simulink model "x35BusNetworkElectricityTransmissionModel"  (R2023b)
settings: Solver=VariableStepAuto  StartTime=0.0  StopTime=0.8  RelTol=1e-3
model workspace (MAT data in the model file):
  Compensation_Ki = 30
  Compensation_Kp = 3
  DC_Ki = 400
  DC_Kp = 8
  F = 0.01
  Flux_min = 0.5
  Grid_Freq_PWM = 2700
  Grid_Ireg_Ki = 5
  Grid_Ireg_Kp = 0.83
  Grid_Ireg_lim = 1.1
  Grid_Modindex_Upper = 1.1
  Grid_conv_Imax = 0.8
  H = 0.685
  Idref_max = 0.9
  Iqref_Tc = 0.3
  Ki_Var = 0.05
  Ki_Vreg = 20
  Ksh = 1.1
  L_pu = 0.3
  Llr = 0.16
  Lls = 0.18
  Lm = 2.9
  Nb_wt = 6
  P_mech = 1080000
  Pitch_Ki = 0
  Pitch_Kp = 150
  Pitch_Max = 27
  Pitch_Tc = 0.01
  Pitch_rate = 10
  Q_Filt = 50
  R_pu = 0.003
  Rotor_Freq_PWM = 1620
  Rotor_Ireg_Ki = 8
  Rotor_Ireg_Kp = 0.6
  Rotor_Ireg_lim = 0.1
  Rotor_Modindex_Upper = 2
  Rr = 0.016
  Rs = 0.023
  T_set = 0.0001
  Tp = 5e-05
  Ts = 5e-06
  Var_C_Filt = 720000
  Var_reg_max = 1.1
  Var_reg_min = 0.9
  WT_Coeff = [0.645 116 0.4 5 21 0.00912 0.08 0.035]
  WT_H = 4.32
  WT_IGBTRon = 5.931
  WT_Param = [91.204 10143]
  Wind_Freq_Filt = 10000
  Wind_Freq_nom = 60
  Wind_P_nom = 1200000
  Wind_Rotor_V_nom = 1950
  Wind_V_nom = 500
  Zeta_Filt = 0.707106781187
  init = [-0.2 0 0 0 0 0 0 0]
  p = 3
  torque0 = 0.83
  v_Ki = 0.1
  v_Kp = 3.6
  v_Max = 1.2
  v_Min = 0.7
  v_T = 5
  vreg_max = 1
  wind_VDC_nom = 1150
  wt0 = 1.2
undefined symbols (not defined in the file): D1, D11, Delta, DiscIntNeverNeededParam, Ion, Lithium, P, Q
libraries: powerlib_extras x144, spsSeriesRLCBranchLib x67, spsLoadFlowBusLib x43, spsThreePhaseTransformerTwoWindingsLib x32, spsThreePhaseSeriesRLCLoadLib x31, spsThreePhaseVIMeasurementLib x26, simulink_extras x26, spsDistributedParametersLineLib x22, spsGenericPowerSystemStabilizerLib x20, spsSynchronousMachinepuStandardLib x10, spsExcitationSystemLib x10, spsHydraulicTurbineandGovernorLib x10
(part 8 of 16)

== system x35BusNetworkElectricityTransmissionModel/400 kV Solar Farm/VSC Control/Current Regulator ==
  VdVq_mes : Inport  PortDimensions=2
  IdIq_mes : Inport  Port=2  PortDimensions=2
  IdIq_ref : Inport  Port=3  PortDimensions=2
  Add1 : Sum  Inputs=++-
  Add2 : Sum
  Add3 : Sum  Inputs=+++
  Demux : Demux  Outputs=2
  Demux1 : Demux  Outputs=2
  Ltot_pu1 : Gain  Gain=Ltot_pu  SaturateOnIntegerOverflow=on  OutDataTypeStr=Inherit: Same as input  ParamDataTypeStr=Inherit: Same as input
  Ltot_pu2 : Gain  Gain=Ltot_pu  SaturateOnIntegerOverflow=on  OutDataTypeStr=Inherit: Same as input  ParamDataTypeStr=Inherit: Same as input
  Mux : Mux  Inputs=2
  PI : slpidlib/PID Controller  Controller=PI  Form=Parallel  TimeDomain=Discrete-time  UseExternalTs=off  SampleTime=Ts  IntegratorMethod=Forward Euler  FilterMethod=Forward Euler  ControllerParametersSource=internal  P=Kp_Ireg  I=Ki_Ireg  UseKiTs=off  D=0  N=100  UseFilter=on  TunerSelectOption=Transfer Function Based (PID Tuner App)  InitialConditionSource=internal  InitialConditionForIntegrator=0  InitialConditionForFilter=0  DifferentiatorICPrevScaledInput=0  ExternalReset=none  TrackingMode=off  Kt=1  LimitOutput=on  SatLimitsSource=internal  UpperSaturationLimit=2  LowerSaturationLimit=-2  LinearizeAsGain=off  AntiWindupMode=none  Kb=1  LimitIntegrator=off  UpperIntegratorSaturationLimit=inf  LowerIntegratorSaturationLimit=-inf  POutMin=[]  POutMax=[]  IOutMin=[]  IOutMax=[]  DOutMin=[]  DOutMax=[]  NOutMin=[]  NOutMax=[]  SumOutMin=[]  SumOutMax=[]  SaturationOutMin=[]  SaturationOutMax=[]  PParamMin=[]  PParamMax=[]  IParamMin=[]  IParamMax=[]  DParamMin=[]  DParamMax=[]  NParamMin=[]  NParamMax=[]  KbParamMin=[]  KbParamMax=[]  KtParamMin=[]  KtParamMax=[]  KbOutMin=[]  KbOutMax=[]  KtOutMin=[]  KtOutMax=[]  IntegratorOutMin=[]  IntegratorOutMax=[]  FilterOutMin=[]  FilterOutMax=[]  SumI1OutMin=[]  SumI1OutMax=[]  SumI2OutMin=[]  SumI2OutMax=[]  SumI3OutMin=[]  SumI3OutMax=[]  SumI4OutMin=[]  SumI4OutMax=[]  SumDOutMin=[]  SumDOutMax=[]  DifferentiatorOutMin=[]  DifferentiatorOutMax=[]  FilterDiffOutCoefMin=[]  FilterDiffOutCoefMax=[]  ReciprocalOutMin=[]  ReciprocalOutMax=[]  SumDenOutMin=[]  SumDenOutMax=[]  SumNumOutMin=[]  SumNumOutMax=[]  DivideOutMin=[]  DivideOutMax=[]  UdiffTsProdOutMin=[]  UdiffTsProdOutMax=[]  NTsProdOutMin=[]  NTsProdOutMax=[]  UintegralTsProdOutMin=[]  UintegralTsProdOutMax=[]  UngainTsProdOutMin=[]  UngainTsProdOutMax=[]  ClampingZeroOutDataTypeStr=Inherit: Inherit via back propagation  ClampingZeroOutMin=[]  ClampingZeroOutMax=[]  FilterDenConstantOutDataTypeStr=Inherit: Inherit via back propagation  FilterDenConstantOutMin=[]  FilterDenConstantOutMax=[]  PCopyOutDataTypeStr=Inherit: Inherit via back propagation  PCopyOutMin=[]  PCopyOutMax=[]  NCopyOutDataTypeStr=Inherit: Inherit via back propagation  NCopyOutMin=[]  NCopyOutMax=[]  IntegratorContinuousStateAttributes=''  IntegratorStateMustResolveToSignalObject=off  IntegratorRTWStateStorageClass=Auto  FilterContinuousStateAttributes=''  FilterStateMustResolveToSignalObject=off  FilterRTWStateStorageClass=Auto  ParallelPVariant=InternalParameters  IdealPVariant=Disabled  IVariant=InternalParameters  DVariant=Disabled  IntegratorVariant=Discrete  SatVariant=Enabled  AWVariant=Passthrough  PCopyVariant=Disabled  TRVariant=Disabled  FdbkBlocksVariant=Forward  IdealPFdbkVariant=Disabled  SatFdbkVariant=Disabled  DerivativeFilterVariant=Disabled  NVariant=Disabled  NCopyVariant=Disabled_SignalSpec  FilterICVariant=Disabled  IntegratorICVariant=InternalICs  ExternalResetVariant=Disabled  TRSumVariant=Passthrough  SumFdbkVariant=Disabled  SumVariant=Sum_PI  TsampFilterVariant=InternalTs  TsampNgainVariant=Passthrough  TsampIntegralVariant=Disabled_SignalSpec  ExternalSaturationOutDataTypeStr=Inherit: Same as second input
  PI_Ireg1 : Scope
  Rtot_pu1 : Gain  Gain=Rtot_pu  SaturateOnIntegerOverflow=on  OutDataTypeStr=Inherit: Same as input  ParamDataTypeStr=Inherit: Same as input
  Rtot_pu5 : Gain  Gain=Rtot_pu  SaturateOnIntegerOverflow=on  OutDataTypeStr=Inherit: Same as input  ParamDataTypeStr=Inherit: Same as input
  Saturation : Saturate  UpperLimit=2  LowerLimit=-2
  Sum : Sum  Inputs=|-+
  VdVq_conv : Outport  VectorParamsAs1DForOutWhenUnconnected=off
  wires:
  Mux/1 -> PI_Ireg1/1, Add2/2
  PI/1 -> Add2/1  "PI"
  Sum/1 -> PI/1
  IdIq_ref/1 -> Sum/2, Demux1/1
  IdIq_mes/1 -> Sum/1
  Add2/1 -> Saturation/1
  Saturation/1 -> VdVq_conv/1
  VdVq_mes/1 -> Demux/1
  Demux/1 -> Add1/1
  Rtot_pu1/1 -> Add1/2
  Demux1/1 -> Rtot_pu1/1, Ltot_pu2/1
  Ltot_pu1/1 -> Add1/3
  Demux1/2 -> Ltot_pu1/1, Rtot_pu5/1
  Rtot_pu5/1 -> Add3/2
  Ltot_pu2/1 -> Add3/3
  Add1/1 -> Mux/1  "Feedforward"
  Demux/2 -> Add3/1
  Add3/1 -> Mux/2

== system x35BusNetworkElectricityTransmissionModel/400 kV Solar Farm/VSC Control/PLL & Measurements ==
  Vabc_prim : Inport
  Iabc_prim : Inport  Port=2
  PLL (3ph) : spsPLL3phLib/PLL (3ph)  Fmin=45  Par_Init="[-0.57  Fnom]"  ParK=[180, 3200, 1]  TcD=Ts  MaxRateChangeFreq=12  FilterCutOffFreq=25  Ts=Ts  AGC=on
  Selector1 : Selector  InputPortWidth=3  IndexOptions=Index vector (dialog)  Indices=[1 2]  OutputSizes=1
  Selector2 : Selector  InputPortWidth=3  IndexOptions=Index vector (dialog)  Indices=[1 2]  OutputSizes=1
  Terminator : Terminator
  V->pu : Gain  Gain=1/(Vnom_prim*sqrt(2)/sqrt(3))  SaturateOnIntegerOverflow=on  OutDataTypeStr=Inherit: Same as input  ParamDataTypeStr=Inherit: Same as input
  V->pu1 : Gain  Gain=Vnom_prim*sqrt(3)/Pnom/sqrt(2)  SaturateOnIntegerOverflow=on  OutDataTypeStr=Inherit: Same as input  ParamDataTypeStr=Inherit: Same as input
  abc to dq0 : spsabctodq0Lib/abc to dq0  Alignment=90 degrees behind phase A axis
  abc to dq1 : spsabctodq0Lib/abc to dq0  Alignment=90 degrees behind phase A axis
  wt : Outport  VectorParamsAs1DForOutWhenUnconnected=off
  VdVq_prim : Outport  Port=2  VectorParamsAs1DForOutWhenUnconnected=off
  IdIq_prim : Outport  Port=3  VectorParamsAs1DForOutWhenUnconnected=off
  wires:
  V->pu1/1 -> abc to dq1/1
  V->pu/1 -> PLL (3ph)/1, abc to dq0/1
  abc to dq1/1 -> Selector1/1
  Vabc_prim/1 -> V->pu/1
  Iabc_prim/1 -> V->pu1/1
  abc to dq0/1 -> Selector2/1
  Selector2/1 -> VdVq_prim/1
  Selector1/1 -> IdIq_prim/1
  PLL (3ph)/2 -> wt/1, abc to dq1/2, abc to dq0/2
  PLL (3ph)/1 -> Terminator/1

== system x35BusNetworkElectricityTransmissionModel/400 kV Solar Farm/VSC Control/Uabc_ref Generation max (m) = 1 ==
  note: (Correction for transformer
      |  D1 connection)
  note: (Correction for delai of Ts_Control)
  wt : Inport
  VdVq_conv : Inport  Port=2
  Add1 : Sum  Inputs=++++
  Add2 : Sum
  Complex to Magnitude-Angle : ComplexToMagnitudeAngle
  Constant : Constant  Value=-pi/6
  Constant1 : Constant  Value=Vnom_dc
  Constant2 : Constant  Value="[ 0  -2*pi/3  2*pi/3  ]"
  Constant3 : Constant  Value=Vnom_sec*sqrt(2)/sqrt(3)
  Constant4 : Constant  Value=Ts*Fnom*(2*pi)
  Demux1 : Demux  Outputs=2
  Gain1 : Gain  Gain=1/2
  Product : Product  Inputs=*/  RndMeth=Zero
  Product1 : Product  Inputs=*/  RndMeth=Zero
  Product2 : Product  Inputs=**  RndMeth=Zero
  Real-Imag to Complex : RealImagToComplex
  Saturation : Saturate  UpperLimit=1  LowerLimit=0
  Trigonometric Function : Trigonometry
  Uabc_ref : Outport  VectorParamsAs1DForOutWhenUnconnected=off
  wires:
  Complex to Magnitude-Angle/1 -> Saturation/1
  Constant1/1 -> Gain1/1
  VdVq_conv/1 -> Product1/1
  Product1/1 -> Demux1/1
  Gain1/1 -> Product/1
  Real-Imag to Complex/1 -> Complex to Magnitude-Angle/1
  Demux1/1 -> Real-Imag to Complex/1
  Demux1/2 -> Real-Imag to Complex/2
  Constant2/1 -> Add1/2
  Constant/1 -> Add1/3
  Constant3/1 -> Product/2
  Product/1 -> Product1/2
  Complex to Magnitude-Angle/2 -> Add2/1
  Add1/1 -> Add2/2
  Add2/1 -> Trigonometric Function/1
  Saturation/1 -> Product2/1
  Trigonometric Function/1 -> Product2/2
  Product2/1 -> Uabc_ref/1
  wt/1 -> Add1/1
  Constant4/1 -> Add1/4

== system x35BusNetworkElectricityTransmissionModel/400 kV Solar Farm/VSC Control/VDC Regulator ==
  Vdc_mes : Inport  PortDimensions=1
  Vdc_ref : Inport  Port=2  PortDimensions=1
  PI : slpidlib/PID Controller  Controller=PI  Form=Parallel  TimeDomain=Discrete-time  UseExternalTs=off  SampleTime=Ts  IntegratorMethod=Trapezoidal  FilterMethod=Forward Euler  ControllerParametersSource=internal  P=Kp_VDCreg  I=Ki_VDCreg  UseKiTs=off  D=0  N=100  UseFilter=on  TunerSelectOption=Transfer Function Based (PID Tuner App)  InitialConditionSource=internal  InitialConditionForIntegrator=0  InitialConditionForFilter=0  DifferentiatorICPrevScaledInput=0  ExternalReset=none  TrackingMode=off  Kt=1  LimitOutput=on  SatLimitsSource=internal  UpperSaturationLimit=1.5  LowerSaturationLimit=-1.5  LinearizeAsGain=off  AntiWindupMode=none  Kb=1  LimitIntegrator=off  UpperIntegratorSaturationLimit=inf  LowerIntegratorSaturationLimit=-inf  POutMin=[]  POutMax=[]  IOutMin=[]  IOutMax=[]  DOutMin=[]  DOutMax=[]  NOutMin=[]  NOutMax=[]  SumOutMin=[]  SumOutMax=[]  SaturationOutMin=[]  SaturationOutMax=[]  PParamMin=[]  PParamMax=[]  IParamMin=[]  IParamMax=[]  DParamMin=[]  DParamMax=[]  NParamMin=[]  NParamMax=[]  KbParamMin=[]  KbParamMax=[]  KtParamMin=[]  KtParamMax=[]  KbOutMin=[]  KbOutMax=[]  KtOutMin=[]  KtOutMax=[]  IntegratorOutMin=[]  IntegratorOutMax=[]  FilterOutMin=[]  FilterOutMax=[]  SumI1OutMin=[]  SumI1OutMax=[]  SumI2OutMin=[]  SumI2OutMax=[]  SumI3OutMin=[]  SumI3OutMax=[]  SumI4OutMin=[]  SumI4OutMax=[]  SumDOutMin=[]  SumDOutMax=[]  DifferentiatorOutMin=[]  DifferentiatorOutMax=[]  FilterDiffOutCoefMin=[]  FilterDiffOutCoefMax=[]  ReciprocalOutMin=[]  ReciprocalOutMax=[]  SumDenOutMin=[]  SumDenOutMax=[]  SumNumOutMin=[]  SumNumOutMax=[]  DivideOutMin=[]  DivideOutMax=[]  UdiffTsProdOutMin=[]  UdiffTsProdOutMax=[]  NTsProdOutMin=[]  NTsProdOutMax=[]  UintegralTsProdOutMin=[]  UintegralTsProdOutMax=[]  UngainTsProdOutMin=[]  UngainTsProdOutMax=[]  ClampingZeroOutDataTypeStr=Inherit: Inherit via back propagation  ClampingZeroOutMin=[]  ClampingZeroOutMax=[]  FilterDenConstantOutDataTypeStr=Inherit: Inherit via back propagation  FilterDenConstantOutMin=[]  FilterDenConstantOutMax=[]  PCopyOutDataTypeStr=Inherit: Inherit via back propagation  PCopyOutMin=[]  PCopyOutMax=[]  NCopyOutDataTypeStr=Inherit: Inherit via back propagation  NCopyOutMin=[]  NCopyOutMax=[]  IntegratorContinuousStateAttributes=''  IntegratorStateMustResolveToSignalObject=off  IntegratorRTWStateStorageClass=Auto  FilterContinuousStateAttributes=''  FilterStateMustResolveToSignalObject=off  FilterRTWStateStorageClass=Auto  ParallelPVariant=InternalParameters  IdealPVariant=Disabled  IVariant=InternalParameters  DVariant=Disabled  IntegratorVariant=Discrete  SatVariant=Enabled  AWVariant=Passthrough  PCopyVariant=Disabled  TRVariant=Disabled  FdbkBlocksVariant=Forward  IdealPFdbkVariant=Disabled  SatFdbkVariant=Disabled  DerivativeFilterVariant=Disabled  NVariant=Disabled  NCopyVariant=Disabled_SignalSpec  FilterICVariant=Disabled  IntegratorICVariant=InternalICs  ExternalResetVariant=Disabled  TRSumVariant=Passthrough  SumFdbkVariant=Disabled  SumVariant=Sum_PI  TsampFilterVariant=InternalTs  TsampNgainVariant=Passthrough  TsampIntegralVariant=Disabled_SignalSpec  ExternalSaturationOutDataTypeStr=Inherit: Same as second input
  Rtot_pu3 : Gain  Gain=1/Vnom_dc  SaturateOnIntegerOverflow=on  OutDataTypeStr=Inherit: Same as input  ParamDataTypeStr=Inherit: Same as input
  Sum : Sum  Inputs=|+-
  Id_ref : Outport  SampleTime=Ts  InitialOutput=0  VectorParamsAs1DForOutWhenUnconnected=off
  wires:
  Sum/1 -> Rtot_pu3/1
  Vdc_mes/1 -> Sum/1
  Vdc_ref/1 -> Sum/2
  Rtot_pu3/1 -> PI/1
  PI/1 -> Id_ref/1

== system x35BusNetworkElectricityTransmissionModel/North Network/Regulators 7/Turbine and Excitation Regulators ==
  pref : Inport
  w : Inport  Port=2
  Pe 0 : Inport  Port=3
  Vref : Inport  Port=4
  Vm : Inport  Port=5
  Add : Sum  Inputs=+-
  Complex to Real-Imag : ComplexToRealImag
  Excitation System : spsExcitationSystemLib/Excitation System  tr=20e-3  reg=[ 300, 0.001 ]  exc=[ 1, 0 ]  tgr=[ 0, 0 ]  damp=[ 0.001, 0.1 ]  sat=[ 0, 0 ]  lim=[ -11.5, 11.5, 0 ]  v0="[1.0  1.28]"
      settings: LibrarySourceBlock=sps_lib/Electrical Machines/Synchronous Machine Control/Excitation System
  Hydraulic Turbine and Governor : spsHydraulicTurbineandGovernorLib/Hydraulic Turbine and Governor  sm="[ 10/3  0.07 ]"  gate="[  0.01  0.97518  -0.1  0.1 ]"  reg="[  0.05  1.163  0.105  0  0.01  ]"  hyd="[  0  2.67  ]"  dref=0  po=0.7516
      settings: LibrarySourceBlock=|
      | sps_lib/Electrical Machines/Synchronous Machine Control/Hydraulic Turbine
      | and Governor
  Stabilitator : Subsystem
  Terminator : Terminator
  wref : Constant
  wref1 : Constant
  Pm : Outport
  Vf : Outport  Port=2
  wires:
  pref/1 -> Hydraulic Turbine and Governor/2
  Complex to Real-Imag/2 -> Excitation System/3
  wref/1 -> Hydraulic Turbine and Governor/1
  Add/1 -> Stabilitator/3(dw), Hydraulic Turbine and Governor/5
  Vm/1 -> Complex to Real-Imag/1
  Pe 0/1 -> Stabilitator/2(Pe), Hydraulic Turbine and Governor/4
  Hydraulic Turbine and Governor/2 -> Terminator/1
  Stabilitator/1(Out1) -> Excitation System/4
  w/1 -> Add/1, Hydraulic Turbine and Governor/3
  Excitation System/1 -> Vf/1
  Hydraulic Turbine and Governor/1 -> Pm/1, Stabilitator/1(Pm)
  Vref/1 -> Excitation System/1
  wref1/1 -> Add/2
  Complex to Real-Imag/1 -> Excitation System/2

== system x35BusNetworkElectricityTransmissionModel/North Network/Regulators 8/Turbine and Excitation Regulators ==
  pref : Inport
  w : Inport  Port=2
  Pe 0 : Inport  Port=3
  Vref : Inport  Port=4
  Vm : Inport  Port=5
  Add : Sum  Inputs=+-
  Complex to Real-Imag : ComplexToRealImag
  Excitation System : spsExcitationSystemLib/Excitation System  tr=20e-3  reg=[ 300, 0.001 ]  exc=[ 1, 0 ]  tgr=[ 0, 0 ]  damp=[ 0.001, 0.1 ]  sat=[ 0, 0 ]  lim=[ -11.5, 11.5, 0 ]  v0="[1.0  1.28]"
      settings: LibrarySourceBlock=sps_lib/Electrical Machines/Synchronous Machine Control/Excitation System
  Hydraulic Turbine and Governor : spsHydraulicTurbineandGovernorLib/Hydraulic Turbine and Governor  sm="[ 10/3  0.07 ]"  gate="[  0.01  0.97518  -0.1  0.1 ]"  reg="[  0.05  1.163  0.105  0  0.01  ]"  hyd="[  0  2.67  ]"  dref=0  po=0.7516
      settings: LibrarySourceBlock=|
      | sps_lib/Electrical Machines/Synchronous Machine Control/Hydraulic Turbine
      | and Governor
  Stabilitator : Subsystem
  Terminator : Terminator
  wref : Constant
  wref1 : Constant
  Pm : Outport
  Vf : Outport  Port=2
  wires:
  pref/1 -> Hydraulic Turbine and Governor/2
  Complex to Real-Imag/2 -> Excitation System/3
  wref/1 -> Hydraulic Turbine and Governor/1
  Add/1 -> Stabilitator/3(dw), Hydraulic Turbine and Governor/5
  Vm/1 -> Complex to Real-Imag/1
  Pe 0/1 -> Stabilitator/2(Pe), Hydraulic Turbine and Governor/4
  Hydraulic Turbine and Governor/2 -> Terminator/1
  Stabilitator/1(Out1) -> Excitation System/4
  w/1 -> Add/1, Hydraulic Turbine and Governor/3
  Excitation System/1 -> Vf/1
  Hydraulic Turbine and Governor/1 -> Pm/1, Stabilitator/1(Pm)
  Vref/1 -> Excitation System/1
  wref1/1 -> Add/2
  Complex to Real-Imag/1 -> Excitation System/2

== system x35BusNetworkElectricityTransmissionModel/North Network/Regulators 9/Turbine and Excitation Regulators ==
  pref : Inport
  w : Inport  Port=2
  Pe 0 : Inport  Port=3
  Vref : Inport  Port=4
  Vm : Inport  Port=5
  Add : Sum  Inputs=+-
  Complex to Real-Imag : ComplexToRealImag
  Excitation System : spsExcitationSystemLib/Excitation System  tr=20e-3  reg=[ 300, 0.001 ]  exc=[ 1, 0 ]  tgr=[ 0, 0 ]  damp=[ 0.001, 0.1 ]  sat=[ 0, 0 ]  lim=[ -11.5, 11.5, 0 ]  v0="[1.0  1.28]"
      settings: LibrarySourceBlock=sps_lib/Electrical Machines/Synchronous Machine Control/Excitation System
  Hydraulic Turbine and Governor : spsHydraulicTurbineandGovernorLib/Hydraulic Turbine and Governor  sm="[ 10/3  0.07 ]"  gate="[  0.01  0.97518  -0.1  0.1 ]"  reg="[  0.05  1.163  0.105  0  0.01  ]"  hyd="[  0  2.67  ]"  dref=0  po=0.7516
      settings: LibrarySourceBlock=|
      | sps_lib/Electrical Machines/Synchronous Machine Control/Hydraulic Turbine
      | and Governor
  Stabilitator : Subsystem
  Terminator : Terminator
  wref : Constant
  wref1 : Constant
  Pm : Outport
  Vf : Outport  Port=2
  wires:
  pref/1 -> Hydraulic Turbine and Governor/2
  Complex to Real-Imag/2 -> Excitation System/3
  wref/1 -> Hydraulic Turbine and Governor/1
  Add/1 -> Stabilitator/3(dw), Hydraulic Turbine and Governor/5
  Vm/1 -> Complex to Real-Imag/1
  Pe 0/1 -> Stabilitator/2(Pe), Hydraulic Turbine and Governor/4
  Hydraulic Turbine and Governor/2 -> Terminator/1
  Stabilitator/1(Stab) -> Excitation System/4
  w/1 -> Add/1, Hydraulic Turbine and Governor/3
  Excitation System/1 -> Vf/1
  Hydraulic Turbine and Governor/1 -> Pm/1, Stabilitator/1(Pm)
  Vref/1 -> Excitation System/1
  wref1/1 -> Add/2
  Complex to Real-Imag/1 -> Excitation System/2

== system x35BusNetworkElectricityTransmissionModel/Regulators 10/Turbine and Excitation Regulators/Stabilitator ==
  Pm : Inport
  Pe : Inport  Port=2
  dw : Inport  Port=3
  Add1 : Sum  Inputs=+-
  Generic Power System Stabilizer : spsGenericPowerSystemStabilizerLib/Generic Power System Stabilizer  Tsensor=30e-3  K=20  Twashout=2  Tleadlag1=[50e-3 20e-3]  Tleadlag2=[3 5.4]  VSlimits=[-0.15 0.15]  Vinit=0  Plot_On=off  MagdB_On=on  FreqRange=logspace(-2,2,500)
      settings: LibrarySourceBlock=|
      | sps_lib/Electrical Machines/Synchronous Machine Control/Generic
      | Power System Stabilizer
  Generic Power System Stabilizer1 : spsGenericPowerSystemStabilizerLib/Generic Power System Stabilizer  Tsensor=30e-3  K=20  Twashout=2  Tleadlag1=[50e-3 20e-3]  Tleadlag2=[3 5.4]  VSlimits=[-0.15 0.15]  Vinit=0  Plot_On=off  MagdB_On=on  FreqRange=logspace(-2,2,500)
      settings: LibrarySourceBlock=|
      | sps_lib/Electrical Machines/Synchronous Machine Control/Generic
      | Power System Stabilizer
  Ground : Ground
  Multiport Switch : MultiPortSwitch  DiagnosticForDefault=None  SaturateOnIntegerOverflow=off  InputSameDT=off
  Out1 : Outport
  wires:
  Pm/1 -> Add1/1
  Generic Power System Stabilizer1/1 -> Multiport Switch/4
  Pe/1 -> Add1/2
  Add1/1 -> Generic Power System Stabilizer/1
  Generic Power System Stabilizer/1 -> Multiport Switch/3
  dw/1 -> Generic Power System Stabilizer1/1
  Ground/1 -> Multiport Switch/2
  [PSS_modes] -> Multiport Switch/1
  Multiport Switch/1 -> Out1/1

== system x35BusNetworkElectricityTransmissionModel/South Network/Regulators 1/Turbine and Excitation Regulators ==
  pref : Inport
  w : Inport  Port=2
  Pe 0 : Inport  Port=3
  Vref : Inport  Port=4
  Vm : Inport  Port=5
  Add : Sum  Inputs=+-
  Complex to Real-Imag : ComplexToRealImag
  Excitation System : spsExcitationSystemLib/Excitation System  tr=20e-3  reg=[ 300, 0.001 ]  exc=[ 1, 0 ]  tgr=[ 0, 0 ]  damp=[ 0.001, 0.1 ]  sat=[ 0, 0 ]  lim=[ -11.5, 11.5, 0 ]  v0="[1.0  1.28]"
      settings: LibrarySourceBlock=sps_lib/Electrical Machines/Synchronous Machine Control/Excitation System
  Hydraulic Turbine and Governor : spsHydraulicTurbineandGovernorLib/Hydraulic Turbine and Governor  sm="[ 10/3  0.07 ]"  gate="[  0.01  0.97518  -0.1  0.1 ]"  reg="[  0.05  1.163  0.105  0  0.01  ]"  hyd="[  0  2.67  ]"  dref=0  po=0.7516
      settings: LibrarySourceBlock=|
      | sps_lib/Electrical Machines/Synchronous Machine Control/Hydraulic Turbine
      | and Governor
  Stabilitator : Subsystem
  Terminator : Terminator
  wref : Constant
  wref1 : Constant
  Pm : Outport
  Vf : Outport  Port=2
  wires:
  pref/1 -> Hydraulic Turbine and Governor/2
  Complex to Real-Imag/2 -> Excitation System/3
  wref/1 -> Hydraulic Turbine and Governor/1
  Add/1 -> Stabilitator/3(dw), Hydraulic Turbine and Governor/5
  Vm/1 -> Complex to Real-Imag/1
  Pe 0/1 -> Stabilitator/2(Pe), Hydraulic Turbine and Governor/4
  Hydraulic Turbine and Governor/2 -> Terminator/1
  Stabilitator/1(Out1) -> Excitation System/4
  w/1 -> Add/1, Hydraulic Turbine and Governor/3
  Excitation System/1 -> Vf/1
  Hydraulic Turbine and Governor/1 -> Pm/1, Stabilitator/1(Pm)
  Vref/1 -> Excitation System/1
  wref1/1 -> Add/2
  Complex to Real-Imag/1 -> Excitation System/2

== system x35BusNetworkElectricityTransmissionModel/South Network/Regulators 2/Turbine and Excitation Regulators ==
  pref : Inport
  w : Inport  Port=2
  Pe 0 : Inport  Port=3
  Vref : Inport  Port=4
  Vm : Inport  Port=5
  Add : Sum  Inputs=+-
  Complex to Real-Imag : ComplexToRealImag
  Excitation System : spsExcitationSystemLib/Excitation System  tr=20e-3  reg=[ 300, 0.001 ]  exc=[ 1, 0 ]  tgr=[ 0, 0 ]  damp=[ 0.001, 0.1 ]  sat=[ 0, 0 ]  lim=[ -11.5, 11.5, 0 ]  v0="[1.0  1.28]"
      settings: LibrarySourceBlock=sps_lib/Electrical Machines/Synchronous Machine Control/Excitation System
  Hydraulic Turbine and Governor : spsHydraulicTurbineandGovernorLib/Hydraulic Turbine and Governor  sm="[ 10/3  0.07 ]"  gate="[  0.01  0.97518  -0.1  0.1 ]"  reg="[  0.05  1.163  0.105  0  0.01  ]"  hyd="[  0  2.67  ]"  dref=0  po=0.7516
      settings: LibrarySourceBlock=|
      | sps_lib/Electrical Machines/Synchronous Machine Control/Hydraulic Turbine
      | and Governor
  Stabilitator : Subsystem
  Terminator : Terminator
  wref : Constant
  wref1 : Constant
  Pm : Outport
  Vf : Outport  Port=2
  wires:
  pref/1 -> Hydraulic Turbine and Governor/2
  Complex to Real-Imag/2 -> Excitation System/3
  wref/1 -> Hydraulic Turbine and Governor/1
  Add/1 -> Stabilitator/3(dw), Hydraulic Turbine and Governor/5
  Vm/1 -> Complex to Real-Imag/1
  Pe 0/1 -> Stabilitator/2(Pe), Hydraulic Turbine and Governor/4
  Hydraulic Turbine and Governor/2 -> Terminator/1
  Stabilitator/1(Out1) -> Excitation System/4
  w/1 -> Add/1, Hydraulic Turbine and Governor/3
  Excitation System/1 -> Vf/1
  Hydraulic Turbine and Governor/1 -> Pm/1, Stabilitator/1(Pm)
  Vref/1 -> Excitation System/1
  wref1/1 -> Add/2
  Complex to Real-Imag/1 -> Excitation System/2

== system x35BusNetworkElectricityTransmissionModel/South Network/Regulators 3/Turbine and Excitation Regulators ==
  pref : Inport
  w : Inport  Port=2
  Pe 0 : Inport  Port=3
  Vref : Inport  Port=4
  Vm : Inport  Port=5
  Add : Sum  Inputs=+-
  Complex to Real-Imag : ComplexToRealImag
  Excitation System : spsExcitationSystemLib/Excitation System  tr=20e-3  reg=[ 300, 0.001 ]  exc=[ 1, 0 ]  tgr=[ 0, 0 ]  damp=[ 0.001, 0.1 ]  sat=[ 0, 0 ]  lim=[ -11.5, 11.5, 0 ]  v0="[1.0  1.28]"
      settings: LibrarySourceBlock=sps_lib/Electrical Machines/Synchronous Machine Control/Excitation System
  Hydraulic Turbine and Governor : spsHydraulicTurbineandGovernorLib/Hydraulic Turbine and Governor  sm="[ 10/3  0.07 ]"  gate="[  0.01  0.97518  -0.1  0.1 ]"  reg="[  0.05  1.163  0.105  0  0.01  ]"  hyd="[  0  2.67  ]"  dref=0  po=0.7516
      settings: LibrarySourceBlock=|
      | sps_lib/Electrical Machines/Synchronous Machine Control/Hydraulic Turbine
      | and Governor
  Stabilitator : Subsystem
  Terminator : Terminator
  wref : Constant
  wref1 : Constant
  Pm : Outport
  Vf : Outport  Port=2
  wires:
  pref/1 -> Hydraulic Turbine and Governor/2
  Complex to Real-Imag/2 -> Excitation System/3
  wref/1 -> Hydraulic Turbine and Governor/1
  Add/1 -> Stabilitator/3(dw), Hydraulic Turbine and Governor/5
  Vm/1 -> Complex to Real-Imag/1
  Pe 0/1 -> Stabilitator/2(Pe), Hydraulic Turbine and Governor/4
  Hydraulic Turbine and Governor/2 -> Terminator/1
  Stabilitator/1(Out1) -> Excitation System/4
  w/1 -> Add/1, Hydraulic Turbine and Governor/3
  Excitation System/1 -> Vf/1
  Hydraulic Turbine and Governor/1 -> Pm/1, Stabilitator/1(Pm)
  Vref/1 -> Excitation System/1
  wref1/1 -> Add/2
  Complex to Real-Imag/1 -> Excitation System/2

== system x35BusNetworkElectricityTransmissionModel/South Network/Regulators 4/Turbine and Excitation Regulators ==
  pref : Inport
  w : Inport  Port=2
  Pe 0 : Inport  Port=3
  Vref : Inport  Port=4
  Vm : Inport  Port=5
  Add : Sum  Inputs=+-
  Complex to Real-Imag : ComplexToRealImag
  Excitation System : spsExcitationSystemLib/Excitation System  tr=20e-3  reg=[ 300, 0.001 ]  exc=[ 1, 0 ]  tgr=[ 0, 0 ]  damp=[ 0.001, 0.1 ]  sat=[ 0, 0 ]  lim=[ -11.5, 11.5, 0 ]  v0="[1.0  1.28]"
      settings: LibrarySourceBlock=sps_lib/Electrical Machines/Synchronous Machine Control/Excitation System
  Hydraulic Turbine and Governor : spsHydraulicTurbineandGovernorLib/Hydraulic Turbine and Governor  sm="[ 10/3  0.07 ]"  gate="[  0.01  0.97518  -0.1  0.1 ]"  reg="[  0.05  1.163  0.105  0  0.01  ]"  hyd="[  0  2.67  ]"  dref=0  po=0.7516
      settings: LibrarySourceBlock=|
      | sps_lib/Electrical Machines/Synchronous Machine Control/Hydraulic Turbine
      | and Governor
  Stabilitator : Subsystem
  Terminator : Terminator
  wref : Constant
  wref1 : Constant
  Pm : Outport
  Vf : Outport  Port=2
  wires:
  pref/1 -> Hydraulic Turbine and Governor/2
  Complex to Real-Imag/2 -> Excitation System/3
  wref/1 -> Hydraulic Turbine and Governor/1
  Add/1 -> Hydraulic Turbine and Governor/5, Stabilitator/3(dw)
  Vm/1 -> Complex to Real-Imag/1
  Pe 0/1 -> Stabilitator/2(Pe), Hydraulic Turbine and Governor/4
  Hydraulic Turbine and Governor/2 -> Terminator/1
  Stabilitator/1(Out1) -> Excitation System/4
  w/1 -> Add/1, Hydraulic Turbine and Governor/3
  Excitation System/1 -> Vf/1
  Hydraulic Turbine and Governor/1 -> Pm/1, Stabilitator/1(Pm)
  Vref/1 -> Excitation System/1
  wref1/1 -> Add/2
  Complex to Real-Imag/1 -> Excitation System/2

== system x35BusNetworkElectricityTransmissionModel/South Network/Regulators 5/Turbine and Excitation Regulators ==
  pref : Inport
  w : Inport  Port=2
  Pe 0 : Inport  Port=3
  Vref : Inport  Port=4
  Vm : Inport  Port=5
  Add : Sum  Inputs=+-
  Complex to Real-Imag : ComplexToRealImag
  Excitation System : spsExcitationSystemLib/Excitation System  tr=20e-3  reg=[ 300, 0.001 ]  exc=[ 1, 0 ]  tgr=[ 0, 0 ]  damp=[ 0.001, 0.1 ]  sat=[ 0, 0 ]  lim=[ -11.5, 11.5, 0 ]  v0="[1.0  1.28]"
      settings: LibrarySourceBlock=sps_lib/Electrical Machines/Synchronous Machine Control/Excitation System
  Hydraulic Turbine and Governor : spsHydraulicTurbineandGovernorLib/Hydraulic Turbine and Governor  sm="[ 10/3  0.07 ]"  gate="[  0.01  0.97518  -0.1  0.1 ]"  reg="[  0.05  1.163  0.105  0  0.01  ]"  hyd="[  0  2.67  ]"  dref=0  po=0.7516
      settings: LibrarySourceBlock=|
      | sps_lib/Electrical Machines/Synchronous Machine Control/Hydraulic Turbine
      | and Governor
  Stabilitator : Subsystem
  Terminator : Terminator
  wref : Constant
  wref1 : Constant
  Pm : Outport
  Vf : Outport  Port=2
  wires:
  pref/1 -> Hydraulic Turbine and Governor/2
  Complex to Real-Imag/2 -> Excitation System/3
  wref/1 -> Hydraulic Turbine and Governor/1
  Add/1 -> Stabilitator/3(dw), Hydraulic Turbine and Governor/5
  Vm/1 -> Complex to Real-Imag/1
  Pe 0/1 -> Stabilitator/2(Pe), Hydraulic Turbine and Governor/4
  Hydraulic Turbine and Governor/2 -> Terminator/1
  Stabilitator/1(Out1) -> Excitation System/4
  w/1 -> Add/1, Hydraulic Turbine and Governor/3
  Excitation System/1 -> Vf/1
  Hydraulic Turbine and Governor/1 -> Pm/1, Stabilitator/1(Pm)
  Vref/1 -> Excitation System/1
  wref1/1 -> Add/2
  Complex to Real-Imag/1 -> Excitation System/2

== system x35BusNetworkElectricityTransmissionModel/South Network/Regulators 6/Turbine and Excitation Regulators ==
  pref : Inport
  w : Inport  Port=2
  Pe 0 : Inport  Port=3
  Vref : Inport  Port=4
  Vm : Inport  Port=5
  Add : Sum  Inputs=+-
  Complex to Real-Imag : ComplexToRealImag
  Excitation System : spsExcitationSystemLib/Excitation System  tr=20e-3  reg=[ 300, 0.001 ]  exc=[ 1, 0 ]  tgr=[ 0, 0 ]  damp=[ 0.001, 0.1 ]  sat=[ 0, 0 ]  lim=[ -11.5, 11.5, 0 ]  v0="[1.0  1.28]"
      settings: LibrarySourceBlock=sps_lib/Electrical Machines/Synchronous Machine Control/Excitation System
  Hydraulic Turbine and Governor : spsHydraulicTurbineandGovernorLib/Hydraulic Turbine and Governor  sm="[ 10/3  0.07 ]"  gate="[  0.01  0.97518  -0.1  0.1 ]"  reg="[  0.05  1.163  0.105  0  0.01  ]"  hyd="[  0  2.67  ]"  dref=0  po=0.7516
      settings: LibrarySourceBlock=|
      | sps_lib/Electrical Machines/Synchronous Machine Control/Hydraulic Turbine
      | and Governor
  Stabilitator : Subsystem
  Terminator : Terminator
  wref : Constant
  wref1 : Constant
  Pm : Outport
  Vf : Outport  Port=2
  wires:
  pref/1 -> Hydraulic Turbine and Governor/2
  Complex to Real-Imag/2 -> Excitation System/3
  wref/1 -> Hydraulic Turbine and Governor/1
  Add/1 -> Stabilitator/3(dw), Hydraulic Turbine and Governor/5
  Vm/1 -> Complex to Real-Imag/1
  Pe 0/1 -> Stabilitator/2(Pe), Hydraulic Turbine and Governor/4
  Hydraulic Turbine and Governor/2 -> Terminator/1
  Stabilitator/1(Out1) -> Excitation System/4
  w/1 -> Add/1, Hydraulic Turbine and Governor/3
  Excitation System/1 -> Vf/1
  Hydraulic Turbine and Governor/1 -> Pm/1, Stabilitator/1(Pm)
  Vref/1 -> Excitation System/1
  wref1/1 -> Add/2
  Complex to Real-Imag/1 -> Excitation System/2

== system x35BusNetworkElectricityTransmissionModel/ 41.4 MW Wind Generation/41.4 MW Wind Farm/10.35 MW Wind Turbine 1/Wind Turbine & Generator 1 ==
  Generator speed (pu) : Inport
  Constant : Constant  Value=14
  Shaft : Subsystem
  Turbine : Subsystem
  "Wind Turbine " : Subsystem  mask{WT_Coeff8=WT_Coeff, WT_Param=WT_Param, vw0=11, Pmech_Out=1.035e7, Ts=Ts}
      mask prompts: WT_Coeff8 "Wind Turbine Coefficients"; WT_Param "Wind Turbine Coefficients"; vw0 "Initial Wind Speed (m/s)"; Pmech_Out "Nominal Mechanical Output Power"; Ts "Sample Time"
  T_shaft (pu) : Outport  VectorParamsAs1DForOutWhenUnconnected=off
  wires:
  [Pitch_WT1] -> "Wind Turbine "/2(Pitch angle (deg))
  Shaft/1(T_shaft (pu)) -> T_shaft (pu)/1, Turbine/2(T_shaft (pu))
  Generator speed (pu)/1 -> Turbine/3(Generator speed (pu))
  Turbine/2(W_wt (pu)) -> "Wind Turbine "/1(Generator speed (pu)1)
  Turbine/1(Turbine speed) -> Shaft/1(Speed)
  Constant/1 -> "Wind Turbine "/3(Wind speed (m/s))
  "Wind Turbine "/1(Tt (pu)) -> Turbine/1(T_wt (pu))

== system x35BusNetworkElectricityTransmissionModel/ 41.4 MW Wind Generation/41.4 MW Wind Farm/10.35 MW Wind Turbine 2/Wind Turbine & Generator 1 ==
  Generator speed (pu) : Inport
  Constant : Constant  Value=14
  Shaft : Subsystem
  Turbine : Subsystem
  "Wind Turbine " : Subsystem  mask{WT_Coeff8=WT_Coeff, WT_Param=WT_Param, vw0=11, Pmech_Out=1.035e7, Ts=Ts}
      mask prompts: WT_Coeff8 "Wind Turbine Coefficients"; WT_Param "Wind Turbine Coefficients"; vw0 "Initial Wind Speed (m/s)"; Pmech_Out "Nominal Mechanical Output Power"; Ts "Sample Time"
  T_shaft (pu) : Outport  VectorParamsAs1DForOutWhenUnconnected=off
  wires:
  [Pitch_WT1] -> "Wind Turbine "/2(Pitch angle (deg))
  Shaft/1(T_shaft (pu)) -> T_shaft (pu)/1, Turbine/2(T_shaft (pu))
  Generator speed (pu)/1 -> Turbine/3(Generator speed (pu))
  Turbine/2(W_wt (pu)) -> "Wind Turbine "/1(Generator speed (pu)1)
  Turbine/1(Turbine speed) -> Shaft/1(Speed)
  Constant/1 -> "Wind Turbine "/3(Wind speed (m/s))
  "Wind Turbine "/1(Tt (pu)) -> Turbine/1(T_wt (pu))

== system x35BusNetworkElectricityTransmissionModel/ 41.4 MW Wind Generation/41.4 MW Wind Farm/10.35 MW Wind Turbine 3/Wind Turbine & Generator 1 ==
  Generator speed (pu) : Inport
  Constant : Constant  Value=14
  Shaft : Subsystem
  Turbine : Subsystem
  "Wind Turbine " : Subsystem  mask{WT_Coeff8=WT_Coeff, WT_Param=WT_Param, vw0=11, Pmech_Out=1.035e7, Ts=Ts}
      mask prompts: WT_Coeff8 "Wind Turbine Coefficients"; WT_Param "Wind Turbine Coefficients"; vw0 "Initial Wind Speed (m/s)"; Pmech_Out "Nominal Mechanical Output Power"; Ts "Sample Time"
  T_shaft (pu) : Outport  VectorParamsAs1DForOutWhenUnconnected=off
  wires:
  [Pitch_WT1] -> "Wind Turbine "/2(Pitch angle (deg))
  Shaft/1(T_shaft (pu)) -> T_shaft (pu)/1, Turbine/2(T_shaft (pu))
  Generator speed (pu)/1 -> Turbine/3(Generator speed (pu))
  Turbine/2(W_wt (pu)) -> "Wind Turbine "/1(Generator speed (pu)1)
  Turbine/1(Turbine speed) -> Shaft/1(Speed)
  Constant/1 -> "Wind Turbine "/3(Wind speed (m/s))
  "Wind Turbine "/1(Tt (pu)) -> Turbine/1(T_wt (pu))

== system x35BusNetworkElectricityTransmissionModel/ 41.4 MW Wind Generation/41.4 MW Wind Farm/10.35 MW Wind Turbine 4/Wind Turbine & Generator 1 ==
  Generator speed (pu) : Inport
  Constant : Constant  Value=14
  Shaft : Subsystem
  Turbine : Subsystem
  "Wind Turbine " : Subsystem  mask{WT_Coeff8=WT_Coeff, WT_Param=WT_Param, vw0=11, Pmech_Out=1.035e7, Ts=Ts}
      mask prompts: WT_Coeff8 "Wind Turbine Coefficients"; WT_Param "Wind Turbine Coefficients"; vw0 "Initial Wind Speed (m/s)"; Pmech_Out "Nominal Mechanical Output Power"; Ts "Sample Time"
  T_shaft (pu) : Outport  VectorParamsAs1DForOutWhenUnconnected=off
  wires:
  [Pitch_WT1] -> "Wind Turbine "/2(Pitch angle (deg))
  Shaft/1(T_shaft (pu)) -> T_shaft (pu)/1, Turbine/2(T_shaft (pu))
  Generator speed (pu)/1 -> Turbine/3(Generator speed (pu))
  Turbine/2(W_wt (pu)) -> "Wind Turbine "/1(Generator speed (pu)1)
  Turbine/1(Turbine speed) -> Shaft/1(Speed)
  Constant/1 -> "Wind Turbine "/3(Wind speed (m/s))
  "Wind Turbine "/1(Tt (pu)) -> Turbine/1(T_wt (pu))

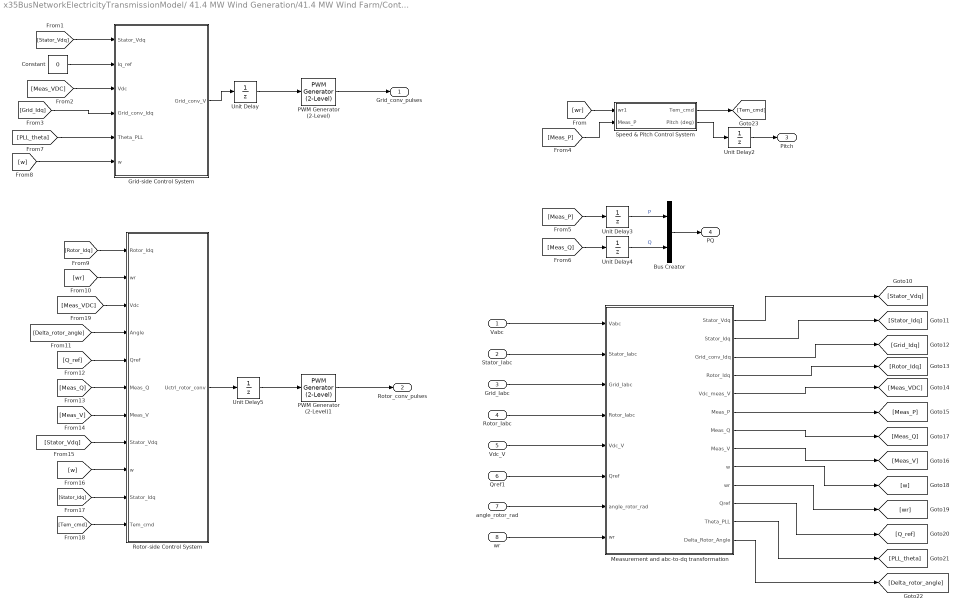
== system x35BusNetworkElectricityTransmissionModel/ 41.4 MW Wind Generation/41.4 MW Wind Farm/Control System/Control System 1 ==
  Vabc : Inport
  Stator_Iabc : Inport  Port=2
  Grid_Iabc : Inport  Port=3
  Rotor_Iabc : Inport  Port=4
  Vdc_V : Inport  Port=5
  Qref1 : Inport  Port=6
  angle_rotor_rad : Inport  Port=7
  wr : Inport  Port=8
  Bus Creator : BusCreator  Inputs=P,Q
  Constant : Constant  Value=0
  Grid-side Control System : Subsystem
  "Measurement and abc-to-dq transformation " : Subsystem
  PWM Generator (2-Level) : spsPWMGenerator2LevelLib/PWM Generator (2-Level)  ModulatorType=Three-phase bridge (6 pulses)  ModulatorMode=Unsynchronized  Fc=Grid_Freq_PWM  Pc=90  nF=27  MinMax="[ -1  1 ]"  SamplingTechnique=Natural  ModulatingSignals=off  m=0.8  Freq=60  Phase=0  Ts=Ts  ShowCarrierOutport=off
  PWM Generator (2-Level)1 : spsPWMGenerator2LevelLib/PWM Generator (2-Level)  ModulatorType=Three-phase bridge (6 pulses)  ModulatorMode=Unsynchronized  Fc=Rotor_Freq_PWM  Pc=90  nF=27  MinMax="[ -1  1 ]"  SamplingTechnique=Natural  ModulatingSignals=off  m=0.8  Freq=60  Phase=0  Ts=Ts  ShowCarrierOutport=off
  Rotor-side Control System : Subsystem
  Speed & Pitch Control System : Subsystem
  Unit Delay{,2..5} (5 alike) : UnitDelay  SampleTime=Ts  HasFrameUpgradeWarning=on
  Grid_conv_pulses : Outport
  Rotor_conv_pulses : Outport  Port=2
  Pitch : Outport  Port=3
  PQ : Outport  Port=4
  wires:
  [Meas_P] -> Speed & Pitch Control System/2(Meas_P)
  "Measurement and abc-to-dq transformation "/1(Stator_Vdq) -> [Stator_Vdq]
  [Meas_Q] -> Unit Delay4/1
  Unit Delay4/1 -> Bus Creator/2  "Q"
  "Measurement and abc-to-dq transformation "/2(Stator_Idq) -> [Stator_Idq]
  "Measurement and abc-to-dq transformation "/9(w) -> [w]
  Grid_Iabc/1 -> "Measurement and abc-to-dq transformation "/3(Grid_Iabc)
  Grid-side Control System/1(Grid_conv_V) -> Unit Delay/1
  Unit Delay5/1 -> PWM Generator (2-Level)1/1
  Unit Delay2/1 -> Pitch/1
  Unit Delay/1 -> PWM Generator (2-Level)/1
  "Measurement and abc-to-dq transformation "/3(Grid_conv_Idq) -> [Grid_Idq]
  Rotor-side Control System/1(Uctrl_rotor_conv) -> Unit Delay5/1
  "Measurement and abc-to-dq transformation "/13(Delta_Rotor_Angle) -> [Delta_rotor_angle]
  PWM Generator (2-Level)/1 -> Grid_conv_pulses/1
  Vabc/1 -> "Measurement and abc-to-dq transformation "/1(Vabc)
  PWM Generator (2-Level)1/1 -> Rotor_conv_pulses/1
  "Measurement and abc-to-dq transformation "/4(Rotor_Idq) -> [Rotor_Idq]
  "Measurement and abc-to-dq transformation "/5(Vdc_meas_V) -> [Meas_VDC]
  angle_rotor_rad/1 -> "Measurement and abc-to-dq transformation "/7(angle_rotor_rad)
  wr/1 -> "Measurement and abc-to-dq transformation "/8(wr)
  "Measurement and abc-to-dq transformation "/7(Meas_Q) -> [Meas_Q]
  Speed & Pitch Control System/2(Pitch (deg)) -> Unit Delay2/1
  Stator_Iabc/1 -> "Measurement and abc-to-dq transformation "/2(Stator_Iabc)
  Speed & Pitch Control System/1(Tem_cmd) -> [Tem_cmd]
  Rotor_Iabc/1 -> "Measurement and abc-to-dq transformation "/4(Rotor_Iabc)
  Vdc_V/1 -> "Measurement and abc-to-dq transformation "/5(Vdc_V)
  Qref1/1 -> "Measurement and abc-to-dq transformation "/6(Qref)
  [wr] -> Speed & Pitch Control System/1(wr1)
  [Meas_P] -> Unit Delay3/1
  Unit Delay3/1 -> Bus Creator/1  "P"
  "Measurement and abc-to-dq transformation "/11("Qref ") -> [Q_ref]
  "Measurement and abc-to-dq transformation "/6(Meas_P) -> [Meas_P]
  "Measurement and abc-to-dq transformation "/12(Theta_PLL) -> [PLL_theta]
  Bus Creator/1 -> PQ/1
  "Measurement and abc-to-dq transformation "/8(Meas_V) -> [Meas_V]
  "Measurement and abc-to-dq transformation "/10("wr ") -> [wr]
  [Stator_Vdq] -> Grid-side Control System/1(Stator_Vdq)
  Constant/1 -> Grid-side Control System/2(Iq_ref)
  [Meas_VDC] -> Grid-side Control System/3(Vdc)
  [Grid_Idq] -> Grid-side Control System/4(Grid_conv_Idq)
  [PLL_theta] -> Grid-side Control System/5(Theta_PLL)
  [w] -> Grid-side Control System/6(w)
  [Rotor_Idq] -> Rotor-side Control System/1(Rotor_Idq)
  [wr] -> Rotor-side Control System/2(wr)
  [Meas_VDC] -> Rotor-side Control System/3(Vdc)
  [Delta_rotor_angle] -> Rotor-side Control System/4(Angle)
  [Q_ref] -> Rotor-side Control System/5(Qref)
  [Meas_Q] -> Rotor-side Control System/6(Meas_Q)
  [Meas_V] -> Rotor-side Control System/7(Meas_V)
  [Stator_Vdq] -> Rotor-side Control System/8(Stator_Vdq)
  [w] -> Rotor-side Control System/9(w)
  [Stator_Idq] -> Rotor-side Control System/10(Stator_Idq)
  [Tem_cmd] -> Rotor-side Control System/11(Tem_cmd)

== system x35BusNetworkElectricityTransmissionModel/ 41.4 MW Wind Generation/41.4 MW Wind Farm/Control System/Control System 2 ==
  Vabc : Inport
  Stator_Iabc : Inport  Port=2
  Grid_Iabc : Inport  Port=3
  Rotor_Iabc : Inport  Port=4
  Vdc_V : Inport  Port=5
  Qref1 : Inport  Port=6
  angle_rotor_rad : Inport  Port=7
  wr : Inport  Port=8
  Bus Creator : BusCreator  Inputs=P,Q
  Constant : Constant  Value=0
  Grid-side Control System : Subsystem
  "Measurement and abc-to-dq transformation " : Subsystem
  PWM Generator (2-Level) : spsPWMGenerator2LevelLib/PWM Generator (2-Level)  ModulatorType=Three-phase bridge (6 pulses)  ModulatorMode=Unsynchronized  Fc=Grid_Freq_PWM  Pc=90  nF=27  MinMax="[ -1  1 ]"  SamplingTechnique=Natural  ModulatingSignals=off  m=0.8  Freq=60  Phase=0  Ts=Ts  ShowCarrierOutport=off
  PWM Generator (2-Level)1 : spsPWMGenerator2LevelLib/PWM Generator (2-Level)  ModulatorType=Three-phase bridge (6 pulses)  ModulatorMode=Unsynchronized  Fc=Rotor_Freq_PWM  Pc=90  nF=27  MinMax="[ -1  1 ]"  SamplingTechnique=Natural  ModulatingSignals=off  m=0.8  Freq=60  Phase=0  Ts=Ts  ShowCarrierOutport=off
  Rotor-side Control System : Subsystem
  Speed & Pitch Control System : Subsystem
  Unit Delay{,2..5} (5 alike) : UnitDelay  SampleTime=Ts  HasFrameUpgradeWarning=on
  Grid_conv_pulses : Outport
  Rotor_conv_pulses : Outport  Port=2
  Pitch : Outport  Port=3
  PQ : Outport  Port=4
  wires:
  [Meas_P] -> Speed & Pitch Control System/2(Meas_P)
  "Measurement and abc-to-dq transformation "/1(Stator_Vdq) -> [Stator_Vdq]
  [Meas_Q] -> Unit Delay4/1
  Unit Delay4/1 -> Bus Creator/2  "Q"
  "Measurement and abc-to-dq transformation "/2(Stator_Idq) -> [Stator_Idq]
  "Measurement and abc-to-dq transformation "/9(w) -> [w]
  Grid_Iabc/1 -> "Measurement and abc-to-dq transformation "/3(Grid_Iabc)
  Grid-side Control System/1(Grid_conv_V) -> Unit Delay/1
  Unit Delay5/1 -> PWM Generator (2-Level)1/1
  Unit Delay2/1 -> Pitch/1
  Unit Delay/1 -> PWM Generator (2-Level)/1
  "Measurement and abc-to-dq transformation "/3(Grid_conv_Idq) -> [Grid_Idq]
  Rotor-side Control System/1(Uctrl_rotor_conv) -> Unit Delay5/1
  "Measurement and abc-to-dq transformation "/13(Delta_Rotor_Angle) -> [Delta_rotor_angle]
  PWM Generator (2-Level)/1 -> Grid_conv_pulses/1
  Vabc/1 -> "Measurement and abc-to-dq transformation "/1(Vabc)
  PWM Generator (2-Level)1/1 -> Rotor_conv_pulses/1
  "Measurement and abc-to-dq transformation "/4(Rotor_Idq) -> [Rotor_Idq]
  "Measurement and abc-to-dq transformation "/5(Vdc_meas_V) -> [Meas_VDC]
  angle_rotor_rad/1 -> "Measurement and abc-to-dq transformation "/7(angle_rotor_rad)
  wr/1 -> "Measurement and abc-to-dq transformation "/8(wr)
  "Measurement and abc-to-dq transformation "/7(Meas_Q) -> [Meas_Q]
  Speed & Pitch Control System/2(Pitch (deg)) -> Unit Delay2/1
  Stator_Iabc/1 -> "Measurement and abc-to-dq transformation "/2(Stator_Iabc)
  Speed & Pitch Control System/1(Tem_cmd) -> [Tem_cmd]
  Rotor_Iabc/1 -> "Measurement and abc-to-dq transformation "/4(Rotor_Iabc)
  Vdc_V/1 -> "Measurement and abc-to-dq transformation "/5(Vdc_V)
  Qref1/1 -> "Measurement and abc-to-dq transformation "/6(Qref)
  [wr] -> Speed & Pitch Control System/1(wr1)
  [Meas_P] -> Unit Delay3/1
  Unit Delay3/1 -> Bus Creator/1  "P"
  "Measurement and abc-to-dq transformation "/11("Qref ") -> [Q_ref]
  "Measurement and abc-to-dq transformation "/6(Meas_P) -> [Meas_P]
  "Measurement and abc-to-dq transformation "/12(Theta_PLL) -> [PLL_theta]
  Bus Creator/1 -> PQ/1
  "Measurement and abc-to-dq transformation "/8(Meas_V) -> [Meas_V]
  "Measurement and abc-to-dq transformation "/10("wr ") -> [wr]
  [Stator_Vdq] -> Grid-side Control System/1(Stator_Vdq)
  Constant/1 -> Grid-side Control System/2(Iq_ref)
  [Meas_VDC] -> Grid-side Control System/3(Vdc)
  [Grid_Idq] -> Grid-side Control System/4(Grid_conv_Idq)
  [PLL_theta] -> Grid-side Control System/5(Theta_PLL)
  [w] -> Grid-side Control System/6(w)
  [Rotor_Idq] -> Rotor-side Control System/1(Rotor_Idq)
  [wr] -> Rotor-side Control System/2(wr)
  [Meas_VDC] -> Rotor-side Control System/3(Vdc)
  [Delta_rotor_angle] -> Rotor-side Control System/4(Angle)
  [Q_ref] -> Rotor-side Control System/5(Qref)
  [Meas_Q] -> Rotor-side Control System/6(Meas_Q)
  [Meas_V] -> Rotor-side Control System/7(Meas_V)
  [Stator_Vdq] -> Rotor-side Control System/8(Stator_Vdq)
  [w] -> Rotor-side Control System/9(w)
  [Stator_Idq] -> Rotor-side Control System/10(Stator_Idq)
  [Tem_cmd] -> Rotor-side Control System/11(Tem_cmd)

== system x35BusNetworkElectricityTransmissionModel/ 41.4 MW Wind Generation/41.4 MW Wind Farm/Control System/Control System 3 ==
  Vabc : Inport
  Stator_Iabc : Inport  Port=2
  Grid_Iabc : Inport  Port=3
  Rotor_Iabc : Inport  Port=4
  Vdc_V : Inport  Port=5
  Qref1 : Inport  Port=6
  angle_rotor_rad : Inport  Port=7
  wr : Inport  Port=8
  Bus Creator : BusCreator  Inputs=P,Q
  Constant : Constant  Value=0
  Grid-side Control System : Subsystem
  "Measurement and abc-to-dq transformation " : Subsystem
  PWM Generator (2-Level) : spsPWMGenerator2LevelLib/PWM Generator (2-Level)  ModulatorType=Three-phase bridge (6 pulses)  ModulatorMode=Unsynchronized  Fc=Grid_Freq_PWM  Pc=90  nF=27  MinMax="[ -1  1 ]"  SamplingTechnique=Natural  ModulatingSignals=off  m=0.8  Freq=60  Phase=0  Ts=Ts  ShowCarrierOutport=off
  PWM Generator (2-Level)1 : spsPWMGenerator2LevelLib/PWM Generator (2-Level)  ModulatorType=Three-phase bridge (6 pulses)  ModulatorMode=Unsynchronized  Fc=Rotor_Freq_PWM  Pc=90  nF=27  MinMax="[ -1  1 ]"  SamplingTechnique=Natural  ModulatingSignals=off  m=0.8  Freq=60  Phase=0  Ts=Ts  ShowCarrierOutport=off
  Rotor-side Control System : Subsystem
  Speed & Pitch Control System : Subsystem
  Unit Delay{,2..5} (5 alike) : UnitDelay  SampleTime=Ts  HasFrameUpgradeWarning=on
  Grid_conv_pulses : Outport
  Rotor_conv_pulses : Outport  Port=2
  Pitch : Outport  Port=3
  PQ : Outport  Port=4
  wires:
  [Meas_P] -> Speed & Pitch Control System/2(Meas_P)
  "Measurement and abc-to-dq transformation "/1(Stator_Vdq) -> [Stator_Vdq]
  [Meas_Q] -> Unit Delay4/1
  Unit Delay4/1 -> Bus Creator/2  "Q"
  "Measurement and abc-to-dq transformation "/2(Stator_Idq) -> [Stator_Idq]
  "Measurement and abc-to-dq transformation "/9(w) -> [w]
  Grid_Iabc/1 -> "Measurement and abc-to-dq transformation "/3(Grid_Iabc)
  Grid-side Control System/1(Grid_conv_V) -> Unit Delay/1
  Unit Delay5/1 -> PWM Generator (2-Level)1/1
  Unit Delay2/1 -> Pitch/1
  Unit Delay/1 -> PWM Generator (2-Level)/1
  "Measurement and abc-to-dq transformation "/3(Grid_conv_Idq) -> [Grid_Idq]
  Rotor-side Control System/1(Uctrl_rotor_conv) -> Unit Delay5/1
  "Measurement and abc-to-dq transformation "/13(Delta_Rotor_Angle) -> [Delta_rotor_angle]
  PWM Generator (2-Level)/1 -> Grid_conv_pulses/1
  Vabc/1 -> "Measurement and abc-to-dq transformation "/1(Vabc)
  PWM Generator (2-Level)1/1 -> Rotor_conv_pulses/1
  "Measurement and abc-to-dq transformation "/4(Rotor_Idq) -> [Rotor_Idq]
  "Measurement and abc-to-dq transformation "/5(Vdc_meas_V) -> [Meas_VDC]
  angle_rotor_rad/1 -> "Measurement and abc-to-dq transformation "/7(angle_rotor_rad)
  wr/1 -> "Measurement and abc-to-dq transformation "/8(wr)
  "Measurement and abc-to-dq transformation "/7(Meas_Q) -> [Meas_Q]
  Speed & Pitch Control System/2(Pitch (deg)) -> Unit Delay2/1
  Stator_Iabc/1 -> "Measurement and abc-to-dq transformation "/2(Stator_Iabc)
  Speed & Pitch Control System/1(Tem_cmd) -> [Tem_cmd]
  Rotor_Iabc/1 -> "Measurement and abc-to-dq transformation "/4(Rotor_Iabc)
  Vdc_V/1 -> "Measurement and abc-to-dq transformation "/5(Vdc_V)
  Qref1/1 -> "Measurement and abc-to-dq transformation "/6(Qref)
  [wr] -> Speed & Pitch Control System/1(wr1)
  [Meas_P] -> Unit Delay3/1
  Unit Delay3/1 -> Bus Creator/1  "P"
  "Measurement and abc-to-dq transformation "/11("Qref ") -> [Q_ref]
  "Measurement and abc-to-dq transformation "/6(Meas_P) -> [Meas_P]
  "Measurement and abc-to-dq transformation "/12(Theta_PLL) -> [PLL_theta]
  Bus Creator/1 -> PQ/1
  "Measurement and abc-to-dq transformation "/8(Meas_V) -> [Meas_V]
  "Measurement and abc-to-dq transformation "/10("wr ") -> [wr]
  [Stator_Vdq] -> Grid-side Control System/1(Stator_Vdq)
  Constant/1 -> Grid-side Control System/2(Iq_ref)
  [Meas_VDC] -> Grid-side Control System/3(Vdc)
  [Grid_Idq] -> Grid-side Control System/4(Grid_conv_Idq)
  [PLL_theta] -> Grid-side Control System/5(Theta_PLL)
  [w] -> Grid-side Control System/6(w)
  [Rotor_Idq] -> Rotor-side Control System/1(Rotor_Idq)
  [wr] -> Rotor-side Control System/2(wr)
  [Meas_VDC] -> Rotor-side Control System/3(Vdc)
  [Delta_rotor_angle] -> Rotor-side Control System/4(Angle)
  [Q_ref] -> Rotor-side Control System/5(Qref)
  [Meas_Q] -> Rotor-side Control System/6(Meas_Q)
  [Meas_V] -> Rotor-side Control System/7(Meas_V)
  [Stator_Vdq] -> Rotor-side Control System/8(Stator_Vdq)
  [w] -> Rotor-side Control System/9(w)
  [Stator_Idq] -> Rotor-side Control System/10(Stator_Idq)
  [Tem_cmd] -> Rotor-side Control System/11(Tem_cmd)
